simulink library "thruster_lib"  (R2016b)
settings: Solver=VariableStepAuto  StartTime=0.0  StopTime=10.0  RelTol=1e-3
undefined symbols (not defined in the file or in its folder): fsw_params, sim_params
libraries: simulink x1
settings Model: Creator=Taylor  LastModifiedBy=Taylor

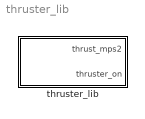
== system thruster_lib ==
  thruster_lib : Subsystem

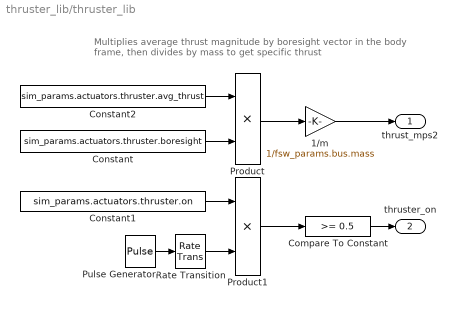
== system thruster_lib/thruster_lib ==
  note: Multiplies average thrust magnitude by boresight vector in the body
      | frame, then divides by mass to get specific thrust
  1/m : Gain  Gain=1/fsw_params.bus.mass
  Compare To Constant : simulink/Logic and Bit Operations/Compare To Constant  relop=>=  const=0.5  OutDataTypeStr=boolean
  Constant : Constant  Value=sim_params.actuators.thruster.boresight  SampleTime=sim_params.sample_time_s
  Constant1 : Constant  Value=sim_params.actuators.thruster.on  OutDataTypeStr=boolean  SampleTime=sim_params.sample_time_s
  Constant2 : Constant  Value=sim_params.actuators.thruster.avg_thrust  SampleTime=sim_params.sample_time_s
  Product : Product
  Product1 : Product
  Pulse Generator : DiscretePulseGenerator  PulseType=Time based  Period=sim_params.CAN.sync_pulse_s  PulseWidth=fsw_params.actuators.pct_sync_pulse
  Rate Transition : RateTransition  OutPortSampleTime=sim_params.sample_time_s
  thrust_mps2 : Outport
  thruster_on : Outport  Port=2
  wires:
  Constant1/1 -> Product1/1
  1/m/1 -> thrust_mps2/1
  Constant/1 -> Product/2
  Constant2/1 -> Product/1
  Product/1 -> 1/m/1
  Pulse Generator/1 -> Rate Transition/1
  Product1/1 -> Compare To Constant/1
  Compare To Constant/1 -> thruster_on/1
  Rate Transition/1 -> Product1/2
